simulink model "FinalProject"  (R2019b)
settings: Solver=FixedStepAuto  StartTime=0.0  StopTime=100  FixedStep=0.01  RelTol=1e-3
undefined symbols (not defined in the file or in its folder): sigbuilder_block
libraries: simulink x1
settings Model: Creator=axs2437  LastModifiedBy=axs2437

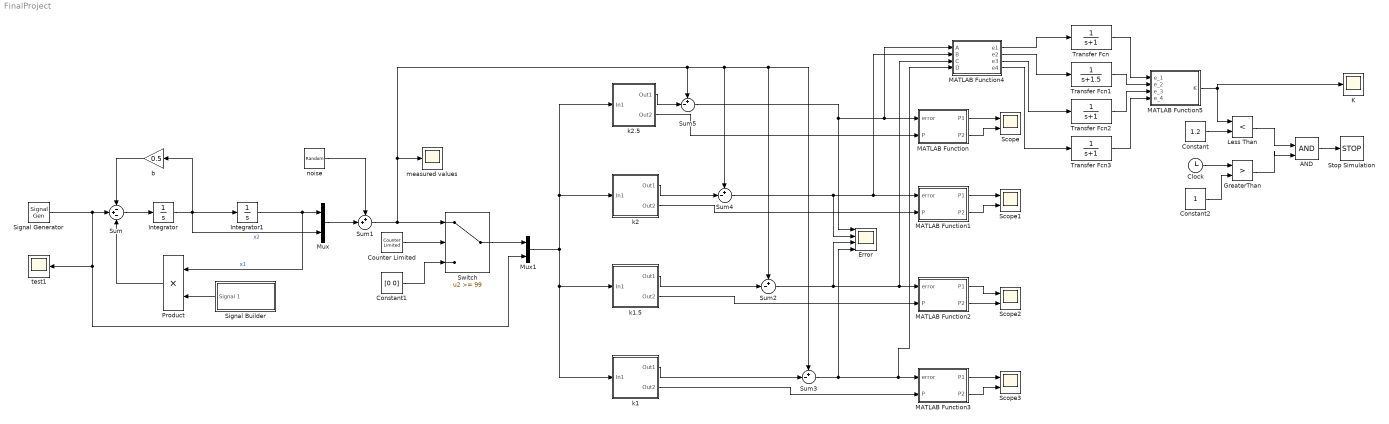
== system FinalProject ==
  AND : Logic  IconShape=distinctive  AllPortsSameDT=off  OutDataTypeStr=boolean
  Clock : Clock
  Constant : Constant  Value=1.2
  Constant1 : Constant  Value=[0 0]
  Constant2 : Constant
  Counter Limited : simulink/Sources/Counter Limited  uplimit=99  tsamp=-1
  Error : Scope  NumInputPorts=4
  GreaterThan : RelationalOperator  Operator=>  OutDataTypeStr=boolean  RndMeth=Simplest
  Integrator : Integrator
  Integrator1 : Integrator
  K : Scope
  Less Than : RelationalOperator  Operator=<  OutDataTypeStr=boolean  RndMeth=Simplest
  MATLAB Function : MATLAB Function  TreatAsAtomicUnit=on
  MATLAB Function1 : MATLAB Function  TreatAsAtomicUnit=on
  MATLAB Function2 : MATLAB Function  TreatAsAtomicUnit=on
  MATLAB Function3 : MATLAB Function  TreatAsAtomicUnit=on
  MATLAB Function4 : MATLAB Function  TreatAsAtomicUnit=on
  MATLAB Function5 : MATLAB Function  TreatAsAtomicUnit=on
  Mux : Mux  Inputs=2
  Mux1 : Mux  Inputs=2
  Product : Product
  Scope{,1..3} (4 alike) : Scope  NumInputPorts=2
  Signal Generator : SignalGenerator  WaveForm=square  Frequency=0.05
  Signal Builder : Subsystem  Tag=STV Subsys  LoadFcn=sigbuilder_block('load');  StartFcn=sigbuilder_block('start');  StopFcn=sigbuilder_block('stop');  ClipboardFcn=sigbuilder_block('clipboard');  mask(Sigbuilder block){tuvar=[0:10]}
      mask help: Simulink:masks:SigbuilderBlock_MD
      mask init:
      | if ~strcmp(get_param(bdroot(gcbh),'SimulationStatus'),'stopped') tuvar = sigbuilder_block('maskInit'); end
      settings: CopyFcn=sigbuilder_block('copy');  DeleteFcn=sigbuilder_block('delete');  ModelCloseFcn=sigbuilder_block('modelClose');  PreSaveFcn=sigbuilder_block('preSave');  PauseFcn=sigbuilder_block('pause');  ContinueFcn=sigbuilder_block('continue');  NameChangeFcn=sigbuilder_block('namechange');  OpenFcn=sigbuilder_block('open',[318.6 104.1 550.2 399.9 ]);  CloseFcn=sigbuilder_block('close');
      mask Display: plot(0, 0, 100, 100,[2, 2, 32, 32, 2], [68, 8, 8, 68, 68],[32, 2], [38, 38], [32, 19, 2],[53, 60, 44], [32, 17, 17, 2],[16, 16, 31, 31]);txt = getActiveGroup(gcbh);text(2, 100, txt,'verticalAlignment', 'top');
  Stop Simulation : Stop
  Sum : Sum  Inputs=-+-
  Sum1 : Sum  Inputs=++|
  Sum{2..5} (4 alike) : Sum  Inputs=+-|
  Switch : Switch  Threshold=99
  Transfer Fcn : TransferFcn  Denominator=[1 1]
  Transfer Fcn1 : TransferFcn  Denominator=[1 1.5]
  Transfer Fcn2 : TransferFcn  Denominator=[1 1]
  Transfer Fcn3 : TransferFcn  Denominator=[1 1]
  b : Gain  Gain=0.5
  k1 : Subsystem
  k1.5 : Subsystem
  k2 : Subsystem
  k2.5 : Subsystem
  measured values : Scope
  noise : RandomNumber  Mean=[0 0]  Variance=[1 1]*0.001  Seed=[5,8]  SampleTime=0.01
  test1 : Scope
  wires:
  Sum/1 -> Integrator/1
  Integrator/1 -> Mux/2, b/1, Integrator1/1  "x2"
  b/1 -> Sum/1
  Integrator1/1 -> Product/1, Mux/1  "x1"
  Mux/1 -> Sum1/2
  Signal Builder/1(Signal 1) -> Product/2
  Product/1 -> Sum/3
  noise/1 -> Sum1/1
  Constant1/1 -> Switch/3
  Counter Limited/1 -> Switch/2
  Signal Generator/1 -> Mux1/2, test1/1, Sum/2
  Switch/1 -> Mux1/1
  Mux1/1 -> k2.5/1(In1), k2/1(In1), k1/1(In1), k1.5/1(In1)
  Sum1/1 -> Switch/1, Sum3/1, Sum2/1, Sum4/1, Sum5/1, measured values/1
  k2.5/1(Out1) -> Sum5/2
  k1/1(Out1) -> Sum3/2
  k1.5/1(Out1) -> Sum2/2
  k2/1(Out1) -> Sum4/2
  Sum5/1 -> MATLAB Function4/1(A), MATLAB Function/1(error), Error/1
  Sum4/1 -> MATLAB Function4/2(B), MATLAB Function1/1(error), Error/2
  Sum2/1 -> MATLAB Function4/3(C), MATLAB Function2/1(error), Error/3
  Sum3/1 -> MATLAB Function4/4(D), MATLAB Function3/1(error), Error/4
  k2.5/2(Out2) -> MATLAB Function/2(P)
  MATLAB Function/1(P1) -> Scope/1
  MATLAB Function/2(P2) -> Scope/2
  k1/2(Out2) -> MATLAB Function3/2(P)
  k1.5/2(Out2) -> MATLAB Function2/2(P)
  k2/2(Out2) -> MATLAB Function1/2(P)
  MATLAB Function3/1(P1) -> Scope3/1
  MATLAB Function3/2(P2) -> Scope3/2
  MATLAB Function2/2(P2) -> Scope2/2
  MATLAB Function2/1(P1) -> Scope2/1
  MATLAB Function1/1(P1) -> Scope1/1
  MATLAB Function1/2(P2) -> Scope1/2
  MATLAB Function4/1(e1) -> Transfer Fcn/1
  MATLAB Function4/2(e2) -> Transfer Fcn1/1
  MATLAB Function4/3(e3) -> Transfer Fcn2/1
  MATLAB Function4/4(e4) -> Transfer Fcn3/1
  Transfer Fcn/1 -> MATLAB Function5/1(e_1)
  Transfer Fcn1/1 -> MATLAB Function5/2(e_2)
  Transfer Fcn2/1 -> MATLAB Function5/3(e_3)
  Transfer Fcn3/1 -> MATLAB Function5/4(e_4)
  MATLAB Function5/1(K) -> K/1, Less Than/1
  Constant/1 -> Less Than/2
  Clock/1 -> GreaterThan/1
  Constant2/1 -> GreaterThan/2
  Less Than/1 -> AND/1
  GreaterThan/1 -> AND/2
  AND/1 -> Stop Simulation/1

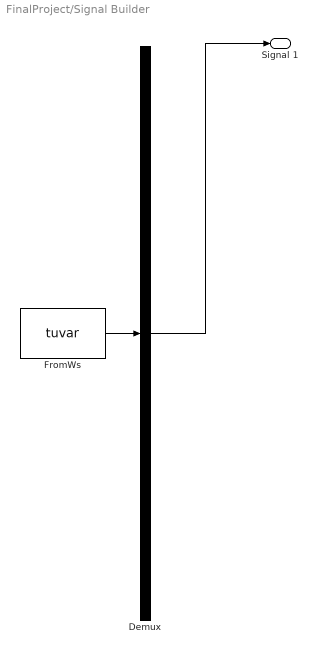
== system FinalProject/Signal Builder ==
  Demux : Demux  Tag=STV Demux  Outputs=1
  FromWs : FromWorkspace  Tag=STV FromWs  VariableName=tuvar  SampleTime=0
      SigBuilderData=|
      | common.afterFinalStr = 'Extrapolate'
      | common.sampleTime = 0
      | dataSet.timeRange = [0 100]
      | dataSet.name = 'Group 1'
      | sbobj.Groups.Name = 'Group 1'
      | sbobj.Groups.Signals.Name = 'Signal 1'
      | sbobj.Groups.Signals.XData = [0 23 23 49 49 75 75 100]
      | sbobj.Groups.Signals.YData = [2.5 2.5 2 2 1.5 1.5 1 1]
      | sbobj.Groups.TimeRange = [0 100]
  Signal 1 : Outport  Tag=STV Outport
  wires:
  Demux/1 -> Signal 1/1
  FromWs/1 -> Demux/1

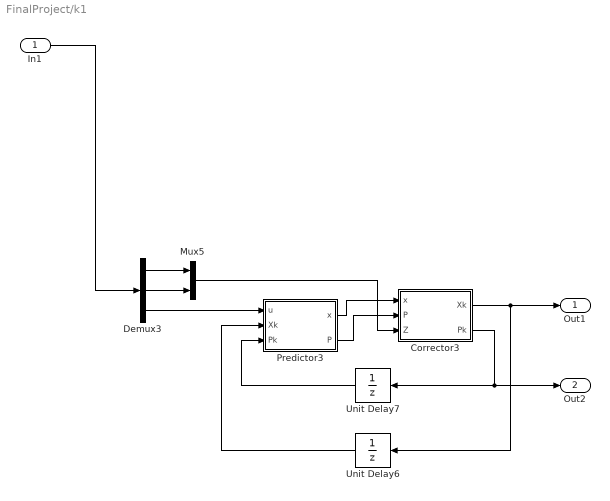
== system FinalProject/k1 ==
  In1 : Inport
  Corrector3 : MATLAB Function  TreatAsAtomicUnit=on
  Demux3 : Demux  Outputs=3
  Mux5 : Mux  Inputs=2
  Predictor3 : MATLAB Function  TreatAsAtomicUnit=on
  Unit Delay6 : UnitDelay  InitialCondition=[0 0]  SampleTime=-1  HasFrameUpgradeWarning=on
  Unit Delay7 : UnitDelay  InitialCondition=eye(2)  SampleTime=-1  HasFrameUpgradeWarning=on
  Out1 : Outport
  Out2 : Outport  Port=2
  wires:
  Mux5/1 -> Corrector3/3(Z)
  Corrector3/2(Pk) -> Unit Delay7/1, Out2/1
  Unit Delay6/1 -> Predictor3/2(Xk)
  Corrector3/1(Xk) -> Out1/1, Unit Delay6/1
  Predictor3/1(x) -> Corrector3/1(x)
  In1/1 -> Demux3/1
  Predictor3/2(P) -> Corrector3/2(P)
  Unit Delay7/1 -> Predictor3/3(Pk)
  Demux3/3 -> Predictor3/1(u)
  Demux3/1 -> Mux5/1
  Demux3/2 -> Mux5/2

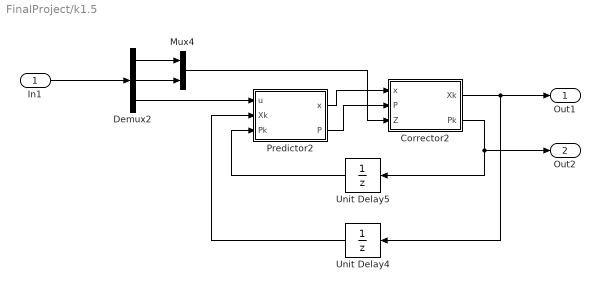
== system FinalProject/k1.5 ==
  In1 : Inport
  Corrector2 : MATLAB Function  TreatAsAtomicUnit=on
  Demux2 : Demux  Outputs=3
  Mux4 : Mux  Inputs=2
  Predictor2 : MATLAB Function  TreatAsAtomicUnit=on
  Unit Delay4 : UnitDelay  InitialCondition=[0 0]  SampleTime=-1  HasFrameUpgradeWarning=on
  Unit Delay5 : UnitDelay  InitialCondition=eye(2)  SampleTime=-1  HasFrameUpgradeWarning=on
  Out1 : Outport
  Out2 : Outport  Port=2
  wires:
  Unit Delay4/1 -> Predictor2/2(Xk)
  Demux2/2 -> Mux4/2
  Predictor2/1(x) -> Corrector2/1(x)
  Demux2/1 -> Mux4/1
  Corrector2/1(Xk) -> Out1/1, Unit Delay4/1
  Unit Delay5/1 -> Predictor2/3(Pk)
  Corrector2/2(Pk) -> Unit Delay5/1, Out2/1
  Demux2/3 -> Predictor2/1(u)
  Predictor2/2(P) -> Corrector2/2(P)
  Mux4/1 -> Corrector2/3(Z)
  In1/1 -> Demux2/1

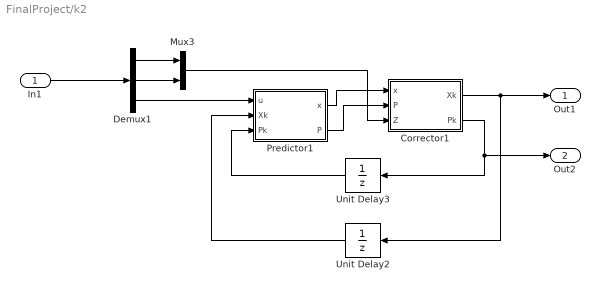
== system FinalProject/k2 ==
  In1 : Inport
  Corrector1 : MATLAB Function  TreatAsAtomicUnit=on
  Demux1 : Demux  Outputs=3
  Mux3 : Mux  Inputs=2
  Predictor1 : MATLAB Function  TreatAsAtomicUnit=on
  Unit Delay2 : UnitDelay  InitialCondition=[0 0]  SampleTime=-1  HasFrameUpgradeWarning=on
  Unit Delay3 : UnitDelay  InitialCondition=eye(2)  SampleTime=-1  HasFrameUpgradeWarning=on
  Out1 : Outport
  Out2 : Outport  Port=2
  wires:
  Demux1/3 -> Predictor1/1(u)
  Corrector1/1(Xk) -> Out1/1, Unit Delay2/1
  Corrector1/2(Pk) -> Unit Delay3/1, Out2/1
  Demux1/2 -> Mux3/2
  Unit Delay2/1 -> Predictor1/2(Xk)
  Predictor1/2(P) -> Corrector1/2(P)
  Demux1/1 -> Mux3/1
  Predictor1/1(x) -> Corrector1/1(x)
  Unit Delay3/1 -> Predictor1/3(Pk)
  Mux3/1 -> Corrector1/3(Z)
  In1/1 -> Demux1/1

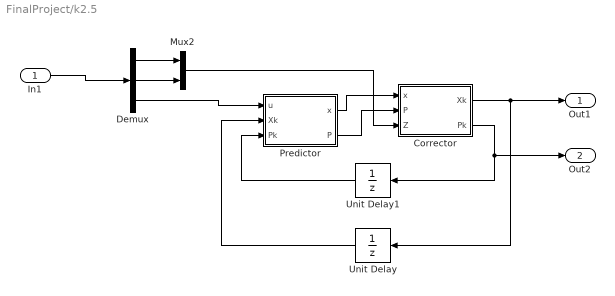
== system FinalProject/k2.5 ==
  In1 : Inport
  Corrector : MATLAB Function  TreatAsAtomicUnit=on
  Demux : Demux  Outputs=3
  Mux2 : Mux  Inputs=2
  Predictor : MATLAB Function  TreatAsAtomicUnit=on
  Unit Delay : UnitDelay  InitialCondition=[0 0]  SampleTime=-1  HasFrameUpgradeWarning=on
  Unit Delay1 : UnitDelay  InitialCondition=eye(2)  SampleTime=-1  HasFrameUpgradeWarning=on
  Out1 : Outport
  Out2 : Outport  Port=2
  wires:
  Mux2/1 -> Corrector/3(Z)
  Corrector/2(Pk) -> Out2/1, Unit Delay1/1
  Predictor/2(P) -> Corrector/2(P)
  Unit Delay1/1 -> Predictor/3(Pk)
  In1/1 -> Demux/1
  Demux/3 -> Predictor/1(u)
  Unit Delay/1 -> Predictor/2(Xk)
  Corrector/1(Xk) -> Out1/1, Unit Delay/1
  Demux/2 -> Mux2/2
  Predictor/1(x) -> Corrector/1(x)
  Demux/1 -> Mux2/1

== matlab function FinalProject/k2.5/Corrector ==
  data: x input; Xk output; P input; Pk output; Z input
function [Xk,Pk] = Corrector(x,P,Z)
H=eye(2); C=eye(2); R=eye(2)/0.01;
if Z(1)==0 && Z(2)==0
    Xk=x;
    Pk=P;
else
    K=P*transpose(H)*inv(H*P*transpose(H)+R);
    Pk=(eye(2)-K*H)*P*transpose(eye(2)-K*H)+K*R*transpose(K);
    Xk=x+K*(Z-H*x);
end
end

== matlab function FinalProject/k2.5/Predictor ==
  data: u input; x output; Xk input; Pk input; P output
function [x,P] = Predictor(u,Xk,Pk)
k=2.5; b=0.5;
A = [0 1;-k -b];
Ae=expm(A*0.01);
B= [0;1];
Bd = (inv(A))*(Ae - eye(2))*B;
Q=eye(2);
F = [-A Q; zeros(2,2) transpose(A)];
G = expm(F*0.01);
Qd=transpose(G(3:4,3:4))*G(1:2,3:4);
x=Ae*Xk + Bd*u;
P=(Ae*Pk*transpose(Ae)+Qd);
end

== matlab function FinalProject/k2/Corrector1 ==
  data: x input; Xk output; P input; Pk output; Z input
function [Xk,Pk] = Corrector(x,P,Z)
H=eye(2); C=eye(2); R=eye(2)/0.01;
if Z(1)==0 && Z(2)==0
    Xk=x;
    Pk=P;
else
    K=P*transpose(H)*inv(H*P*transpose(H)+R);
    Pk=(eye(2)-K*H)*P*transpose(eye(2)-K*H)+K*R*transpose(K);
    Xk=x+K*(Z-H*x);
end
end

== matlab function FinalProject/k2/Predictor1 ==
  data: u input; x output; Xk input; Pk input; P output
function [x,P] = Predictor(u,Xk,Pk)
k=2; b=0.5;
A = [0 1;-k -b];
Ae=expm(A*0.01);
B= [0;1];
Bd = (inv(A))*(Ae - eye(2))*B;
Q=eye(2);
F = [-A Q; zeros(2,2) transpose(A)];
G = expm(F*0.01);
Qd=transpose(G(3:4,3:4))*G(1:2,3:4);
x=Ae*Xk + Bd*u;
P=(Ae*Pk*transpose(Ae)+Qd);
end

== matlab function FinalProject/k1.5/Corrector2 ==
  data: x input; Xk output; P input; Pk output; Z input
function [Xk,Pk] = Corrector(x,P,Z)
H=eye(2); C=eye(2); R=eye(2)/0.01;
if Z(1)==0 && Z(2)==0
    Xk=x;
    Pk=P;
else
    K=P*transpose(H)*inv(H*P*transpose(H)+R);
    Pk=(eye(2)-K*H)*P*transpose(eye(2)-K*H)+K*R*transpose(K);
    Xk=x+K*(Z-H*x);
end
end

== matlab function FinalProject/k1.5/Predictor2 ==
  data: u input; x output; Xk input; Pk input; P output
function [x,P] = Predictor(u,Xk,Pk)
k=1.5; b=0.5;
A = [0 1;-k -b];
Ae=expm(A*0.01);
B= [0;1];
Bd = (inv(A))*(Ae - eye(2))*B;
Q=eye(2);
F = [-A Q; zeros(2,2) transpose(A)];
G = expm(F*0.01);
Qd=transpose(G(3:4,3:4))*G(1:2,3:4);
x=Ae*Xk + Bd*u;
P=(Ae*Pk*transpose(Ae)+Qd);
end

== matlab function FinalProject/k1/Corrector3 ==
  data: x input; Xk output; P input; Pk output; Z input
function [Xk,Pk] = Corrector(x,P,Z)
H=eye(2); C=eye(2); R=eye(2)/0.01;
if Z(1)==0 && Z(2)==0
    Xk=x;
    Pk=P;
else
    K=P*transpose(H)*inv(H*P*transpose(H)+R);
    Pk=(eye(2)-K*H)*P*transpose(eye(2)-K*H)+K*R*transpose(K);
    Xk=x+K*(Z-H*x);
end
end

== matlab function FinalProject/k1/Predictor3 ==
  data: u input; x output; Xk input; Pk input; P output
function [x,P] = Predictor(u,Xk,Pk)
k=1; b=0.5;
A = [0 1;-k -b];
Ae=expm(A*0.01);
B= [0;1];
Bd = (inv(A))*(Ae - eye(2))*B;
Q=eye(2);
F = [-A Q; zeros(2,2) transpose(A)];
G = expm(F*0.01);
Qd=transpose(G(3:4,3:4))*G(1:2,3:4);
x=Ae*Xk + Bd*u;
P=(Ae*Pk*transpose(Ae)+Qd);
end

== matlab function FinalProject/MATLAB Function ==
  data: error input; P1 output; P input; P2 output
function [P1,P2]=covariance(error,P)
P1=[error(1) sqrt(P(1,1)) -sqrt(P(1,1))];
P2=[error(2) sqrt(P(2,2)) -sqrt(P(2,2))];
end

== matlab function FinalProject/MATLAB Function1 ==
  data: error input; P1 output; P input; P2 output
function [P1,P2]=covariance(error,P)
P1=[error(1) sqrt(P(1,1)) -sqrt(P(1,1))];
P2=[error(2) sqrt(P(2,2)) -sqrt(P(2,2))];
end

== matlab function FinalProject/MATLAB Function2 ==
  data: error input; P1 output; P input; P2 output
function [P1,P2]=covariance(error,P)
P1=[error(1) sqrt(P(1,1)) -sqrt(P(1,1))];
P2=[error(2) sqrt(P(2,2)) -sqrt(P(2,2))];
end

== matlab function FinalProject/MATLAB Function3 ==
  data: error input; P1 output; P input; P2 output
function [P1,P2]=covariance(error,P)
P1=[error(1) sqrt(P(1,1)) -sqrt(P(1,1))];
P2=[error(2) sqrt(P(2,2)) -sqrt(P(2,2))];
end

== matlab function FinalProject/MATLAB Function4 ==
  data: A input; e1 output; B input; C input; D input; e2 output; e3 output; e4 output
function [e1,e2,e3,e4] = errorblock(A,B,C,D)
e1=sqrt(A(1)^2+A(2)^2);
e2=sqrt(B(1)^2+B(2)^2);
e3=sqrt(C(1)^2+C(2)^2);
e4=sqrt(D(1)^2+D(2)^2);
end

== matlab function FinalProject/MATLAB Function5 ==
  data: e_1 input; K output; e_2 input; e_3 input; e_4 input
function K = k_estimator(e_1,e_2,e_3,e_4)
[i,j]=min([e_1,e_2,e_3,e_4]);
K=2.5;
switch j
    case 1
        K=2.5;
    case 2
        K=2;
    case 3
        K=1.5;
    case 4
        K=1;
end
